simulink model "BLDC_Trapezoidal_Control"  (R2019a)
settings: Solver=VariableStepAuto  StartTime=0.0  StopTime=20  RelTol=1e-3  AbsTol=1e-3  EnableMultiTasking=on
undefined symbols (not defined in the file): sigbuilder_block
libraries: nesl_utility x14, ee_lib x12, fl_lib x8, simulink x3, powerlib_meascontrol x1
settings Model: Creator=hp  LastModifiedBy=hp
settings SolverCC: AutoScaleAbsTol=off
settings DataIOCC: LimitDataPoints=on  MaxDataPoints=10000
settings OptimizationCC: LifeSpan=inf
settings DebuggingCC: AllowSymbolicDim=off  PregeneratedLibrarySubsystemCodeDiagnostic=none  SFUnexpectedBacktrackingDiag=warning  SFNoUnconditionalDefaultTransitionDiag=warning  SFExecutionAtInitializationDiag=none  ArithmeticOperatorsInVariantConditions=warning
settings SFSimCC: SimUseLocalCustomCode=off
settings RTWCC: RTWUseLocalCustomCode=off
settings CodeAppCC: StateflowObjectComments=on
settings GRTTargetCC: TargetLangStandard=C89/C90 (ANSI)  GeneratePreprocessorConditionals=Disable all
settings ConfigComp: CovMetricSettings=dw  CovHtmlReporting=on  CovSaveCumulativeToWorkspaceVar=on  CovSaveSingleToWorkspaceVar=on  CovExternalEMLEnable=off  CovSFcnEnable=off
settings SimscapeCC: SimscapeLogType=all  SimscapeLogDataHistory=10000

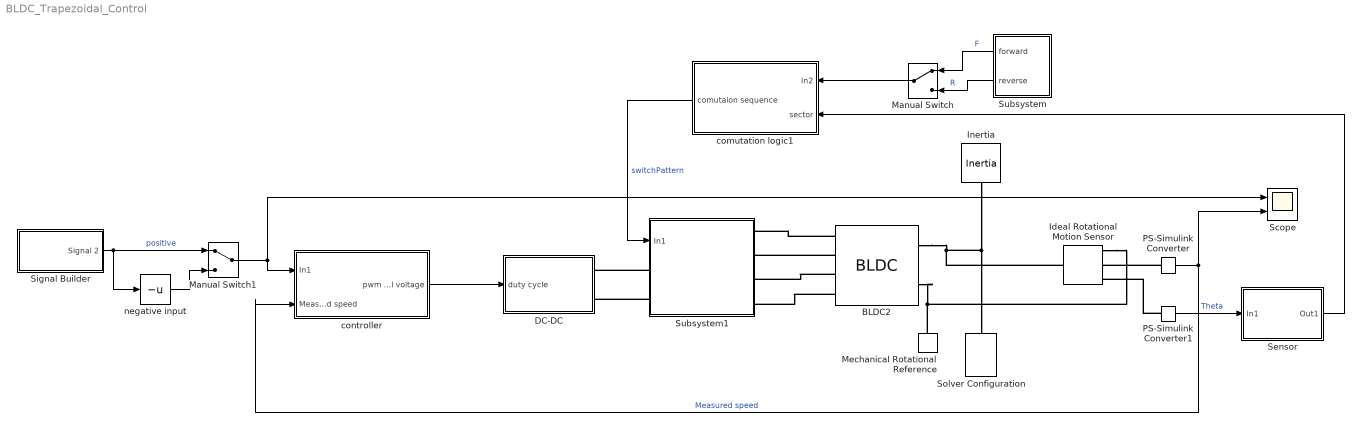
== system BLDC_Trapezoidal_Control ==
  BLDC2 : ee_lib/Electromechanical/Permanent Magnet/BLDC  rotor_param=1  pm_flux_linkage=0.5513 Wb  theta_constant=120/1 deg  emf_max=9.6 V  DphiDtheta_tab=[0, -.1528, -.1528, .1528, .1528, 0] Wb/rad  back_emf_tab=[0, -9.6, -9.6, 9.6, 9.6, 0] V  rotor_angle_tab=[0, 7.5, 22.5, 37.5, 52.5, 60] deg  w_meas=600 rpm  nPolePairs=1  stator_param=2  Ld=0.00022 H  Lq=0.00022 H  L0=0.00016 H  Ls=0.0002 H  Lm=0 H  Ms=0.00002 H  Rs=0.013 Ohm  zero_sequence=ee.enum.park.zerosequence.include  J=0.0001 kg*m^2  lam=0.2 N*m/(rad/s)  axes_param=1  i_d_specify=off  i_d_priority=None  i_d=0 A  i_d_nominal_specify=off  i_d_nominal_unit=A  i_d_nominal_value=1  i_q_specify=off  i_q_priority=None  i_q=0 A  i_q_nominal_specify=off  i_q_nominal_unit=A  i_q_nominal_value=1  torque_specify=off  torque_priority=None  torque=0 N*m  torque_nominal_specify=off  torque_nominal_unit=N*m  torque_nominal_value=1  angular_velocity_specify=off  angular_velocity_priority=High  angular_velocity=0 rpm  angular_velocity_nominal_specify=off  angular_velocity_nominal_unit=rpm  angular_velocity_nominal_value=1  angular_position_specify=off  angular_position_priority=High  angular_position=0 deg  angular_position_nominal_specify=off  angular_position_nominal_unit=deg  angular_position_nominal_value=1
      settings: SourceProductName=Simscape Electrical  SourceProductBaseCode=PS
  "DC-DC " : Subsystem
  Ideal Rotational Motion Sensor : fl_lib/Mechanical/Mechanical Sensors/Ideal Rotational Motion Sensor  offset=0 deg
  Inertia : fl_lib/Mechanical/Rotational Elements/Inertia  inertia=10 kg*m^2  w_specify=off  w_priority=High  w=0 rad/s  w_nominal_specify=off  w_nominal_unit=rad/s  w_nominal_value=1  t_specify=off  t_priority=None  t=0 N*m  t_nominal_specify=off  t_nominal_unit=N*m  t_nominal_value=1
  Manual Switch : ManualSwitch
  Manual Switch1 : ManualSwitch
  Mechanical Rotational Reference : fl_lib/Mechanical/Rotational Elements/Mechanical Rotational Reference
  PS-Simulink Converter : nesl_utility/PS-Simulink Converter  PhysicalDomain=network_engine_domain  SubClassName=ps_output  LeftPortType=input  RightPortType=output  PseudoPeriodic=off  Frequencies=[]  Unit=rpm  AffineConversion=off
  PS-Simulink Converter1 : nesl_utility/PS-Simulink Converter  PhysicalDomain=network_engine_domain  SubClassName=ps_output  LeftPortType=input  RightPortType=output  PseudoPeriodic=off  Frequencies=[]  Unit=deg  AffineConversion=off
  Scope : Scope  NumInputPorts=2
  Sensor : Subsystem
  Signal Builder : Subsystem  Tag=STV Subsys  LoadFcn=sigbuilder_block('load');  StartFcn=sigbuilder_block('start');  StopFcn=sigbuilder_block('stop');  ClipboardFcn=sigbuilder_block('clipboard');  mask(Sigbuilder block){tuvar=[0:10]}
      mask help: Simulink:masks:SigbuilderBlock_MD
      mask init:
      | if ~strcmp(get_param(bdroot(gcbh),'SimulationStatus'),'stopped') tuvar = sigbuilder_block('maskInit'); end
      settings: CopyFcn=sigbuilder_block('copy');  DeleteFcn=sigbuilder_block('delete');  ModelCloseFcn=sigbuilder_block('modelClose');  PreSaveFcn=sigbuilder_block('preSave');  PauseFcn=sigbuilder_block('pause');  ContinueFcn=sigbuilder_block('continue');  NameChangeFcn=sigbuilder_block('namechange');  OpenFcn=sigbuilder_block('open',[6 30 1012.5 447.75 ]);  CloseFcn=sigbuilder_block('close');
      mask Display: plot(0, 0, 100, 100,[2, 2, 32, 32, 2], [68, 8, 8, 68, 68],[32, 2], [38, 38], [32, 19, 2],[53, 60, 44], [32, 17, 17, 2],[16, 16, 31, 31]);txt = getActiveGroup(gcbh);text(2, 100, txt,'verticalAlignment', 'top');
  Solver Configuration : nesl_utility/Solver Configuration  PhysicalDomain=network_engine_domain  SubClassName=solver  LeftPortType=input  RightPortType=generic  Tones=[]  Harmonics=[]  SimulateNoise=off  Profile=off  UseLocalSampling=off  EnableSwitchedLinearOptims=on  FrequencyDomain=off  UseCCode=off  RelTol=0.001  AbsTol=1e-06  MinStep=1e-09  ToWorkspace=off  RevertToSquareIcSolve=off  NumHomotopyIterations=100  PhasorMode=off  PhasorModeNumHarmonics=1  DoDC=off  ResidualTolerance=1e-09  UseLocalSolver=on  LocalSolverChoice=NE_BACKWARD_EULER_ADVANCER  LocalSolverSampleTime=2e-6  DoFixedCost=on  MaxNonlinIter=3  MaxModeIter=2  LinearAlgebra=auto  EquationFormulation=NE_TIME_EF  DelaysMemoryBudget=1024  AutomaticFiltering=on  FilteringTimeConstant=0.001  PartitionStorageMethod=AS_NEEDED  PartitionMemoryBudget=1024  PartitionMethod=ROBUST
  Subsystem : Subsystem
  Subsystem1 : Subsystem
  comutation logic1 : Subsystem
  controller : Subsystem
  negative input : UnaryMinus
  wires:
  comutation logic1/1("comutaion sequence ") -> Subsystem1/1(In1)  "switchPattern"
  PS-Simulink Converter1/1 -> Sensor/1(In1)  "Theta"
  PS-Simulink Converter/1 -> Scope/2, controller/2(Measured speed)  "Measured speed"
  Sensor/1(Out1) -> comutation logic1/2(sector)
  Signal Builder/1(Signal 2) -> negative input/1, Manual Switch1/1  "positive"
  controller/1(pwm control voltage) -> "DC-DC "/1(duty cycle)
  Manual Switch/1 -> comutation logic1/1(In2)
  Subsystem/1(forward) -> Manual Switch/1  "F"
  Subsystem/2(reverse) -> Manual Switch/2  "R"
  negative input/1 -> Manual Switch1/2
  Manual Switch1/1 -> Scope/1, controller/1(In1)
  connections:
  Mechanical Rotational Reference/LConn1 -- BLDC2/RConn2 -- Ideal Rotational Motion Sensor/RConn1
  Inertia/LConn1 -- Solver Configuration/RConn1 -- Ideal Rotational Motion Sensor/LConn1 -- BLDC2/RConn1
  BLDC2/LConn1 -- Subsystem1/RConn1
  BLDC2/LConn2 -- Subsystem1/RConn2
  BLDC2/LConn3 -- Subsystem1/RConn3
  BLDC2/LConn4 -- Subsystem1/RConn4
  PS-Simulink Converter/LConn1 -- Ideal Rotational Motion Sensor/RConn2
  PS-Simulink Converter1/LConn1 -- Ideal Rotational Motion Sensor/RConn3
  Subsystem1/LConn1 -- "DC-DC "/RConn1
  Subsystem1/LConn2 -- "DC-DC "/RConn2

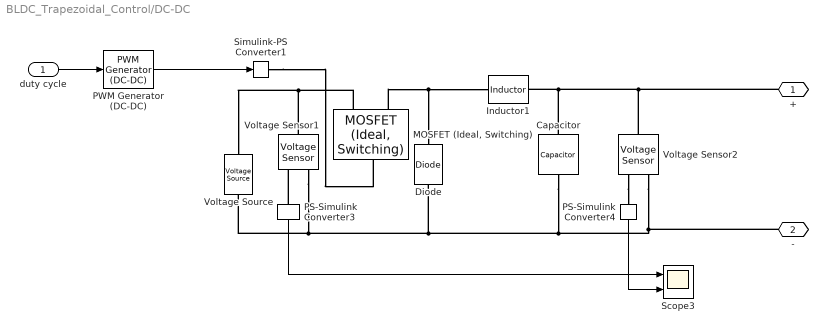
== system BLDC_Trapezoidal_Control/DC-DC  ==
  duty cycle : Inport
  Capacitor : fl_lib/Electrical/Electrical Elements/Capacitor  c=.001 F  r=.2 Ohm  g=0 1/Ohm  i_specify=off  i_priority=None  i=0 A  i_nominal_specify=off  i_nominal_unit=A  i_nominal_value=1  v_specify=off  v_priority=None  v=0 V  v_nominal_specify=off  v_nominal_unit=V  v_nominal_value=1  vc_specify=off  vc_priority=High  vc=0 V  vc_nominal_specify=off  vc_nominal_unit=V  vc_nominal_value=1
  Diode : ee_lib/Semiconductors & Converters/Diode  ModelType=ee.enum.diode.modelType.pwl  Vf=0.6 V  Ron=0.3 Ohm  Goff=1e-8 S  prmExp=ee.enum.diode.expParam.useTwo  I12=[.0137, .545] A  V12=[.6, .7] V  IS=1e-12 A  ec=1  I1=0.0137 A  V1=0.6 V  RS=0 Ohm  Tmeas=25 degC  N_series=1  N_parallel=1  Rz=0.3 Ohm  BV=inf V  C_param=ee.enum.diode.capParam.fixed  CJ=5 pF  CJ0=5 pF  VJ=1 V  Mgrad=0.5  Vvec=[.1, 10, 100] V  Cvec=[3.5, 1, .4] pF  FC=0.5  Q_param=ee.enum.diode.recoveryParam.off  iRM=-7.15 A  iF=4 A  didt=-750 A/us  trr_factor=3  trr=115 ns  Qrr=1500 s*uA  TT=50 ns  tau=100 ns  T_param=ee.enum.diode.temperatureParam.off  IS_T2=1.25e-7 A  I1_T2=0.245 A  V1_T2=0.5 V  Tmeas2=125 degC  EG_param=ee.enum.diode.egapParam.material_si  EG=1.11 eV  XTI_param=ee.enum.diode.xtiParam.pn  XTI=3  dBVdT=0 V/K  Tdevice=25 degC  i_specify=off  i_priority=None  i=0 A  i_nominal_specify=off  i_nominal_unit=A  i_nominal_value=1  v_specify=off  v_priority=None  v=0 V  v_nominal_specify=off  v_nominal_unit=V  v_nominal_value=1  i_capacitor_specify=off  i_capacitor_priority=None  i_capacitor=0 A  i_capacitor_nominal_specify=off  i_capacitor_nominal_unit=A  i_capacitor_nominal_value=1  v_capacitor_specify=off  v_capacitor_priority=None  v_capacitor=0 V  v_capacitor_nominal_specify=off  v_capacitor_nominal_unit=V  v_capacitor_nominal_value=1  power_dissipated_specify=off  power_dissipated_priority=None  power_dissipated=0 W  power_dissipated_nominal_specify=off  power_dissipated_nominal_unit=W  power_dissipated_nominal_value=1  Rth=[0, 10] K/W  thermal_mass_parameterization=ee.enum.thermalNetwork.timeconstant  thermal_mass=[0, 1] J/K  thermal_time_constant=[0, 10] s  thermal_mass_initial_temperatures=[25, 25] degC
      settings: SourceProductName=Simscape Electrical
  Inductor1 : fl_lib/Electrical/Electrical Elements/Inductor  l=.1 H  r=.1 Ohm  g=1e-9 1/Ohm  i_specify=off  i_priority=None  i=0 A  i_nominal_specify=off  i_nominal_unit=A  i_nominal_value=1  v_specify=off  v_priority=None  v=0 V  v_nominal_specify=off  v_nominal_unit=V  v_nominal_value=1  i_L_specify=off  i_L_priority=High  i_L=0 A  i_L_nominal_specify=off  i_L_nominal_unit=A  i_L_nominal_value=1
  "MOSFET (Ideal, Switching)" : ee_lib/Semiconductors & Converters/MOSFET (Ideal, Switching)  Rds=1e-4 Ohm  Goff=1e-6 1/Ohm  Vth=0.5 V  diode_param=2  diode_Vf=.1 V  diode_Ron=0.001 Ohm  diode_Goff=1e-5 1/Ohm  diode_C=50e-9 F  diode_iRM=-235 A  diode_iF=300 A  diode_idot=-50 A/us  diode_trr_param=1  diode_trr_factor=3  diode_trr=15 us  diode_Qrr=1500 s*uA  thermal_loss_option=2  Voff=300 V  Tau=1e-4 s  Tj=[298.15, 398.15] K  Iout_scalar=600 A  Eon_scalar=22.86e-3 J  Eoff_scalar=17.14e-3 J  Von_scalar=2.7 V  Iout_data=[0, 10, 50, 100, 200, 400, 600] A  Eon_data=[0, .29, 1.43, 2.86, 5.71, 13.14, 22.86; 0, .57, 2.63, 5.14, 10.29, 20.57, 30.29] * 1e-3 J  Eoff_data=[0, .21, 1.07, 2.14, 4.29, 9.86, 17.14; 0, .43, 1.97, 3.86, 7.71, 15.43, 22.71] * 1e-3 J  Von_data=[0, 1.1, 1.3, 1.45, 1.75, 2.25, 2.7; 0, 1, 1.15, 1.35, 1.7, 2.35, 3] V
      settings: SourceProductName=Simscape Electrical
  PS-Simulink Converter3 : nesl_utility/PS-Simulink Converter  PhysicalDomain=network_engine_domain  SubClassName=ps_output  LeftPortType=input  RightPortType=output  PseudoPeriodic=off  Frequencies=[]  Unit=1  AffineConversion=off
  PS-Simulink Converter4 : nesl_utility/PS-Simulink Converter  PhysicalDomain=network_engine_domain  SubClassName=ps_output  LeftPortType=input  RightPortType=output  PseudoPeriodic=off  Frequencies=[]  Unit=1  AffineConversion=off
  PWM Generator (DC-DC) : powerlib_meascontrol/Pulse & Signal Generators/PWM Generator (DC-DC)  Fsw=1000  Ts=0
      settings: SourceProductName=Simscape Electrical
  Scope3 : Scope  NumInputPorts=2
  Simulink-PS Converter1 : nesl_utility/Simulink-PS Converter  PhysicalDomain=network_engine_domain  SubClassName=ps_input  LeftPortType=input  RightPortType=output  PseudoPeriodic=off  Frequencies=[]  NoiseDistribution=none  NoiseParameters=[]  Unit=V  AffineConversion=off  FilteringAndDerivatives=provide  SimscapeFilterOrder=1  InputFilterTimeConstant=0.001  UdotUserProvided=0
  Voltage Sensor1 : fl_lib/Electrical/Electrical Sensors/Voltage Sensor
  Voltage Sensor2 : fl_lib/Electrical/Electrical Sensors/Voltage Sensor
  Voltage Source : ee_lib/Sources/Voltage Source  dc_voltage=500 V  ac_voltage=0 V  ac_shift=0 rad  ac_frequency=60 Hz  noise_mode=0  PSD=0 V^2/Hz  repeatability=1  auto_seed=387260031  user_seed=0  sample_time=1e-3 s  i_specify=off  i_priority=None  i=0 A  i_nominal_specify=off  i_nominal_unit=A  i_nominal_value=1  v_specify=off  v_priority=None  v=0 V  v_nominal_specify=off  v_nominal_unit=V  v_nominal_value=1
      settings: SourceProductName=Simscape Electrical
  + : PMIOPort  Side=Right
  - : PMIOPort  Port=2  Side=Right
  wires:
  PWM Generator (DC-DC)/1 -> Simulink-PS Converter1/1
  duty cycle/1 -> PWM Generator (DC-DC)/1
  PS-Simulink Converter4/1 -> Scope3/2
  PS-Simulink Converter3/1 -> Scope3/1
  connections:
  "MOSFET (Ideal, Switching)"/RConn1 -- Voltage Source/LConn1 -- Voltage Sensor1/LConn1
  Voltage Source/RConn1 -- Voltage Sensor2/RConn2 -- -/RConn1 -- Capacitor/RConn1 -- Diode/LConn1 -- Voltage Sensor1/RConn2
  Simulink-PS Converter1/RConn1 -- "MOSFET (Ideal, Switching)"/LConn1
  "MOSFET (Ideal, Switching)"/RConn2 -- Inductor1/LConn1 -- Diode/RConn1
  Capacitor/LConn1 -- +/RConn1 -- Voltage Sensor2/LConn1 -- Inductor1/RConn1
  Voltage Sensor2/RConn1 -- PS-Simulink Converter4/LConn1
  PS-Simulink Converter3/LConn1 -- Voltage Sensor1/RConn1

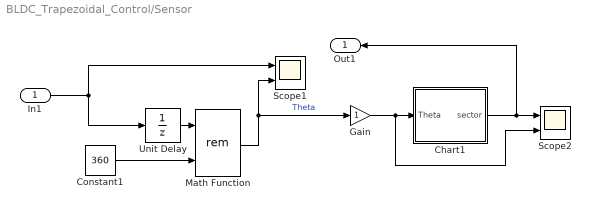
== system BLDC_Trapezoidal_Control/Sensor ==
  In1 : Inport
  Chart1 : Stateflow chart  BlockKeywords=__PRM__SERIALIZED__DATA__:Stateflow Chart,Stateflow Diagram  TreatAsAtomicUnit=on
  Constant1 : Constant  Value=360
  Gain : Gain
  Math Function : Math  Operator=rem  SaturateOnIntegerOverflow=on
  Scope1 : Scope  NumInputPorts=2
  Scope2 : Scope  NumInputPorts=2
  Unit Delay : UnitDelay  SampleTime=-1  HasFrameUpgradeWarning=on
  Out1 : Outport
  wires:
  Chart1/1(sector) -> Out1/1, Scope2/1
  Constant1/1 -> Math Function/2
  Unit Delay/1 -> Math Function/1
  In1/1 -> Scope1/1, Unit Delay/1
  Math Function/1 -> Gain/1, Scope1/2  "Theta"
  Gain/1 -> Chart1/1(Theta), Scope2/2

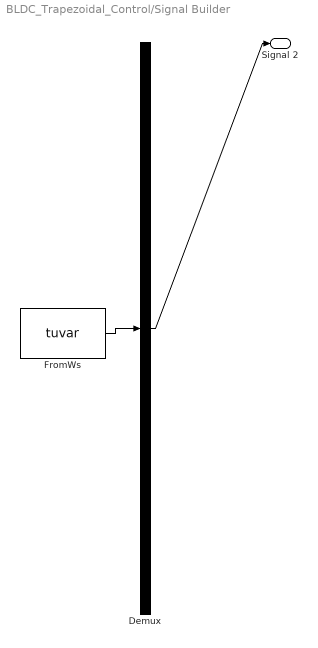
== system BLDC_Trapezoidal_Control/Signal Builder ==
  Demux : Demux  Tag=STV Demux  Outputs=1
  FromWs : FromWorkspace  Tag=STV FromWs  VariableName=tuvar  SampleTime=0
      SigBuilderData=|
      | common.afterFinalStr = 'Extrapolate'
      | common.sampleTime = 0
      | dataSet.timeRange = [0 15]
      | dataSet.name = 'Group 1'
      | sbobj.Groups.Name = 'Group 1'
      | sbobj.Groups.Signals.Name = 'Signal 2'
      | sbobj.Groups.Signals.XData = [0 1.66666666667 3.33333333333 5 6.66666666667 8.33333333333 10 11.6666666667 13.3333333333 15]
      | sbobj.Groups.Signals.YData = [0 270 510 520 780 1000 1000 1380 1500 1510]
      | sbobj.Groups.TimeRange = [0 15]
  Signal 2 : Outport  Tag=STV Outport
  wires:
  FromWs/1 -> Demux/1
  Demux/1 -> Signal 2/1

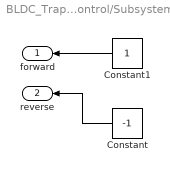
== system BLDC_Trapezoidal_Control/Subsystem ==
  Constant : Constant  Value=-1
  Constant1 : Constant
  forward : Outport
  reverse : Outport  Port=2
  wires:
  Constant/1 -> reverse/1
  Constant1/1 -> forward/1

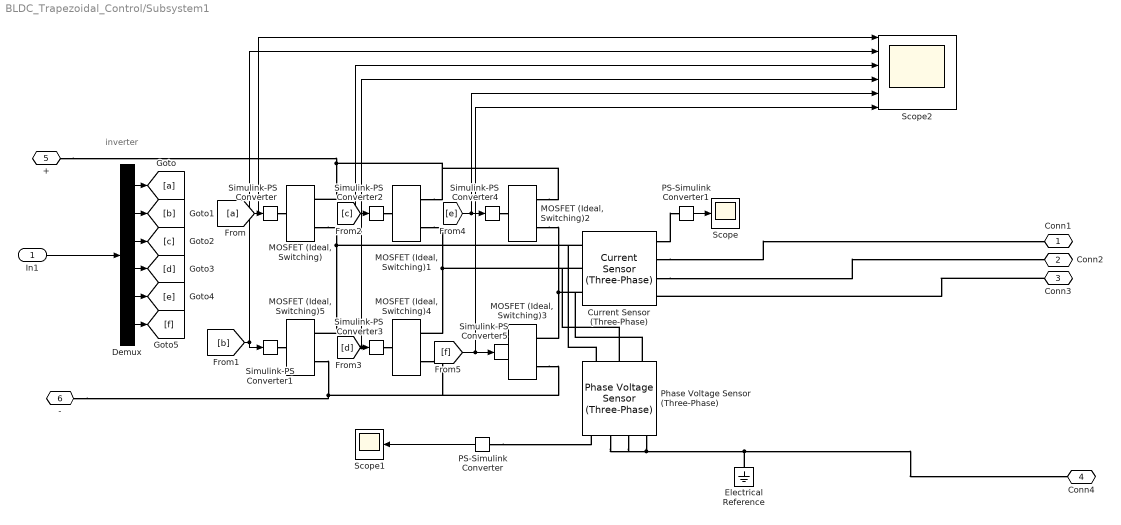
== system BLDC_Trapezoidal_Control/Subsystem1 ==
  note: inverter
  In1 : Inport
  Current Sensor (Three-Phase) : ee_lib/Sensors & Transducers/Current Sensor (Three-Phase)
      settings: SourceProductName=Simscape Electrical
  Demux : Demux  Outputs=6
  Electrical Reference : fl_lib/Electrical/Electrical Elements/Electrical Reference
  MOSFET (Ideal, Switching){,1..5} (6 alike) : ee_lib/Semiconductors & Converters/MOSFET (Ideal, Switching)  Rds=0.01 Ohm  Goff=1e-6 1/Ohm  Vth=.5 V  diode_param=2  diode_Vf=.1 V  diode_Ron=0.001 Ohm  diode_Goff=1e-5 1/Ohm  diode_C=50e-9 F  diode_iRM=-235 A  diode_iF=300 A  diode_idot=-50 A/us  diode_trr_param=1  diode_trr_factor=3  diode_trr=15 us  diode_Qrr=1500 s*uA  thermal_loss_option=2  Voff=300 V  Tau=1e-4 s  Tj=[298.15, 398.15] K  Iout_scalar=600 A  Eon_scalar=22.86e-3 J  Eoff_scalar=17.14e-3 J  Von_scalar=2.7 V  Iout_data=[0, 10, 50, 100, 200, 400, 600] A  Eon_data=[0, .29, 1.43, 2.86, 5.71, 13.14, 22.86; 0, .57, 2.63, 5.14, 10.29, 20.57, 30.29] * 1e-3 J  Eoff_data=[0, .21, 1.07, 2.14, 4.29, 9.86, 17.14; 0, .43, 1.97, 3.86, 7.71, 15.43, 22.71] * 1e-3 J  Von_data=[0, 1.1, 1.3, 1.45, 1.75, 2.25, 2.7; 0, 1, 1.15, 1.35, 1.7, 2.35, 3] V
      settings: SourceProductName=Simscape Electrical
  PS-Simulink Converter : nesl_utility/PS-Simulink Converter  PhysicalDomain=network_engine_domain  SubClassName=ps_output  LeftPortType=input  RightPortType=output  PseudoPeriodic=off  Frequencies=[]  Unit=1  AffineConversion=off
  PS-Simulink Converter1 : nesl_utility/PS-Simulink Converter  PhysicalDomain=network_engine_domain  SubClassName=ps_output  LeftPortType=input  RightPortType=output  PseudoPeriodic=off  Frequencies=[]  Unit=1  AffineConversion=off
  Phase Voltage Sensor (Three-Phase) : ee_lib/Sensors & Transducers/Phase Voltage Sensor (Three-Phase)
      settings: SourceProductName=Simscape Electrical  SourceProductBaseCode=PS
  Scope : Scope
  Scope1 : Scope
  Scope2 : Scope  NumInputPorts=6
  Simulink-PS Converter{,1..5} (6 alike) : nesl_utility/Simulink-PS Converter  PhysicalDomain=network_engine_domain  SubClassName=ps_input  LeftPortType=input  RightPortType=output  PseudoPeriodic=off  Frequencies=[]  NoiseDistribution=none  NoiseParameters=[]  Unit=1  AffineConversion=off  FilteringAndDerivatives=provide  SimscapeFilterOrder=1  InputFilterTimeConstant=0.001  UdotUserProvided=0
  Conn1 : PMIOPort  Side=Right
  Conn2 : PMIOPort  Port=2  Side=Right
  Conn3 : PMIOPort  Port=3  Side=Right
  Conn4 : PMIOPort  Port=4  Side=Right
  + : PMIOPort  Port=5  Side=Left
  - : PMIOPort  Port=6  Side=Left
  wires:
  [c] -> Scope2/3, Simulink-PS Converter2/1
  PS-Simulink Converter1/1 -> Scope/1
  [d] -> Simulink-PS Converter3/1, Scope2/4
  Demux/5 -> [e]
  Demux/3 -> [c]
  Demux/2 -> [b]
  Demux/4 -> [d]
  [f] -> Scope2/6, Simulink-PS Converter5/1
  [e] -> Scope2/5, Simulink-PS Converter4/1
  Demux/1 -> [a]
  Demux/6 -> [f]
  PS-Simulink Converter/1 -> Scope1/1
  [b] -> Scope2/2, Simulink-PS Converter1/1
  In1/1 -> Demux/1
  [a] -> Scope2/1, Simulink-PS Converter/1
  connections:
  "MOSFET (Ideal, Switching)2"/RConn1 -- "MOSFET (Ideal, Switching)1"/RConn1 -- +/RConn1 -- "MOSFET (Ideal, Switching)"/RConn1
  Simulink-PS Converter4/RConn1 -- "MOSFET (Ideal, Switching)2"/LConn1
  Electrical Reference/LConn1 -- Conn4/RConn1 -- Phase Voltage Sensor (Three-Phase)/RConn2 -- Phase Voltage Sensor (Three-Phase)/RConn3 -- Phase Voltage Sensor (Three-Phase)/RConn4
  "MOSFET (Ideal, Switching)1"/RConn2 -- Phase Voltage Sensor (Three-Phase)/LConn2 -- Current Sensor (Three-Phase)/LConn2 -- "MOSFET (Ideal, Switching)4"/RConn1
  "MOSFET (Ideal, Switching)"/RConn2 -- Phase Voltage Sensor (Three-Phase)/LConn1 -- Current Sensor (Three-Phase)/LConn1 -- "MOSFET (Ideal, Switching)5"/RConn1
  Simulink-PS Converter5/RConn1 -- "MOSFET (Ideal, Switching)3"/LConn1
  Simulink-PS Converter1/RConn1 -- "MOSFET (Ideal, Switching)5"/LConn1
  Current Sensor (Three-Phase)/RConn1 -- PS-Simulink Converter1/LConn1
  "MOSFET (Ideal, Switching)5"/RConn2 -- -/RConn1 -- "MOSFET (Ideal, Switching)3"/RConn2 -- "MOSFET (Ideal, Switching)4"/RConn2
  Current Sensor (Three-Phase)/RConn2 -- Conn1/RConn1
  Simulink-PS Converter2/RConn1 -- "MOSFET (Ideal, Switching)1"/LConn1
  Simulink-PS Converter3/RConn1 -- "MOSFET (Ideal, Switching)4"/LConn1
  "MOSFET (Ideal, Switching)2"/RConn2 -- Phase Voltage Sensor (Three-Phase)/LConn3 -- Current Sensor (Three-Phase)/LConn3 -- "MOSFET (Ideal, Switching)3"/RConn1
  PS-Simulink Converter/LConn1 -- Phase Voltage Sensor (Three-Phase)/RConn1
  Simulink-PS Converter/RConn1 -- "MOSFET (Ideal, Switching)"/LConn1
  Current Sensor (Three-Phase)/RConn3 -- Conn2/RConn1
  Conn3/RConn1 -- Current Sensor (Three-Phase)/RConn4

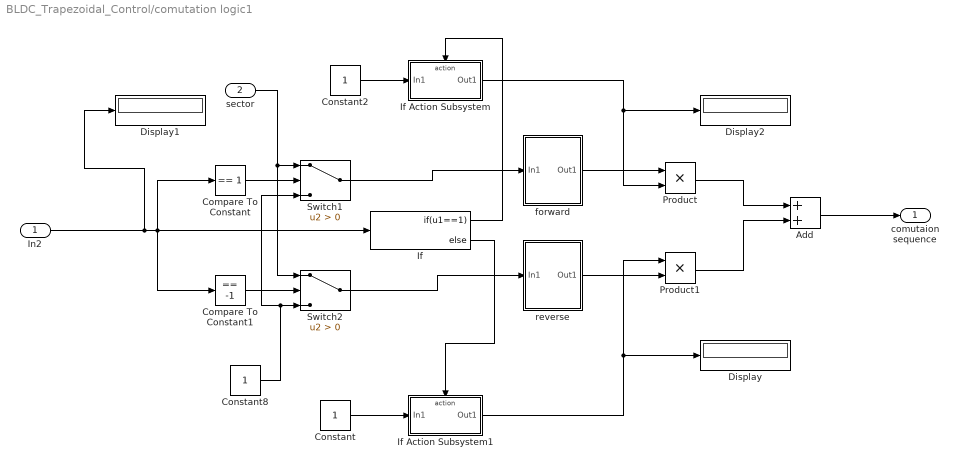
== system BLDC_Trapezoidal_Control/comutation logic1 ==
  In2 : Inport
  sector : Inport  Port=2
  Add : Sum
  Compare To Constant : simulink/Logic and Bit Operations/Compare To Constant  relop===  const=1  OutDataTypeStr=boolean
  Compare To Constant1 : simulink/Logic and Bit Operations/Compare To Constant  relop===  const=-1  OutDataTypeStr=boolean
  Constant : Constant
  Constant2 : Constant
  Constant8 : Constant
  Display : Display
  Display1 : Display
  Display2 : Display
  If : If  IfExpression=u1==1
  If Action Subsystem : Subsystem  TreatAsAtomicUnit=on
  If Action Subsystem1 : Subsystem  TreatAsAtomicUnit=on
  Product : Product
  Product1 : Product
  Switch1 : Switch  Criteria=u2 > Threshold
  Switch2 : Switch  Criteria=u2 > Threshold
  forward : Subsystem
  reverse : Subsystem
  "comutaion sequence " : Outport
  wires:
  In2/1 -> Display1/1, Compare To Constant/1, If/1, Compare To Constant1/1
  Compare To Constant/1 -> Switch1/2
  Compare To Constant1/1 -> Switch2/2
  sector/1 -> Switch2/1, Switch1/1
  Constant8/1 -> Switch1/3, Switch2/3
  Switch1/1 -> forward/1(In1)
  Switch2/1 -> reverse/1(In1)
  Add/1 -> "comutaion sequence "/1
  If/2 -> If Action Subsystem1/Action
  If/1 -> If Action Subsystem/Action
  forward/1(Out1) -> Product/1
  reverse/1(Out1) -> Product1/2
  Product1/1 -> Add/2
  Product/1 -> Add/1
  If Action Subsystem/1(Out1) -> Display2/1, Product/2
  If Action Subsystem1/1(Out1) -> Product1/1, Display/1
  Constant/1 -> If Action Subsystem1/1(In1)
  Constant2/1 -> If Action Subsystem/1(In1)

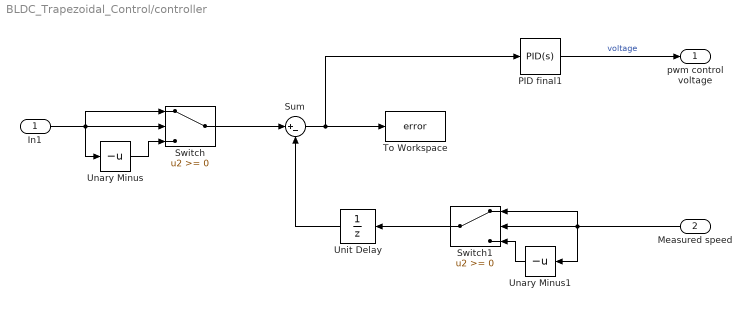
== system BLDC_Trapezoidal_Control/controller ==
  In1 : Inport
  Measured speed : Inport  Port=2
  PID final1 : simulink/Continuous/PID Controller  Controller=PID  Form=Parallel  TimeDomain=Continuous-time  SampleTime=-1  IntegratorMethod=Forward Euler  FilterMethod=Forward Euler  ControllerParametersSource=internal  P=.1  I=.03  D=.01  UseFilter=on  N=100  TunerSelectOption=Transfer Function Based (PID Tuner App)  InitialConditionSource=internal  InitialConditionForIntegrator=0  InitialConditionForFilter=0  DifferentiatorICPrevScaledInput=0  ExternalReset=none  TrackingMode=off  Kt=1  LimitOutput=on  UpperSaturationLimit=1  LowerSaturationLimit=0  LinearizeAsGain=on  AntiWindupMode=clamping  Kb=1  POutMin=[]  POutMax=[]  IOutMin=[]  IOutMax=[]  DOutMin=[]  DOutMax=[]  NOutMin=[]  NOutMax=[]  SumOutMin=[]  SumOutMax=[]  SaturationOutMin=[]  SaturationOutMax=[]  PParamMin=[]  PParamMax=[]  IParamMin=[]  IParamMax=[]  DParamMin=[]  DParamMax=[]  NParamMin=[]  NParamMax=[]  KbParamMin=[]  KbParamMax=[]  KtParamMin=[]  KtParamMax=[]  KbOutMin=[]  KbOutMax=[]  KtOutMin=[]  KtOutMax=[]  IntegratorOutMin=[]  IntegratorOutMax=[]  FilterOutMin=[]  FilterOutMax=[]  SumI1OutMin=[]  SumI1OutMax=[]  SumI2OutMin=[]  SumI2OutMax=[]  SumI3OutMin=[]  SumI3OutMax=[]  SumI4OutMin=[]  SumI4OutMax=[]  SumDOutMin=[]  SumDOutMax=[]  DifferentiatorOutMin=[]  DifferentiatorOutMax=[]  FilterDiffOutCoefMin=[]  FilterDiffOutCoefMax=[]  ReciprocalOutMin=[]  ReciprocalOutMax=[]  SumDenOutMin=[]  SumDenOutMax=[]  SumNumOutMin=[]  SumNumOutMax=[]  DivideOutMin=[]  DivideOutMax=[]  IntegratorContinuousStateAttributes=''  IntegratorStateMustResolveToSignalObject=off  IntegratorRTWStateStorageClass=Auto  FilterContinuousStateAttributes=''  FilterStateMustResolveToSignalObject=off  FilterRTWStateStorageClass=Auto  ParallelPVariant=InternalParameters  IdealPVariant=Disabled  IVariant=InternalParameters  DVariant=InternalParameters  IntegratorVariant=Continuous  SatVariant=Enabled  AWVariant=ContClampingParallel  PCopyVariant=Disabled  TRVariant=Disabled  FdbkBlocksVariant=Forward  IdealPFdbkVariant=Disabled  SatFdbkVariant=Disabled  DerivativeFilterVariant=ContFilter  NVariant=InternalParameters  NCopyVariant=Disabled  FilterICVariant=InternalICsFilter  IntegratorICVariant=InternalICs  ExternalResetVariant=Disabled  TRSumVariant=Passthrough  SumFdbkVariant=Disabled  SumVariant=Sum_PID
  Sum : Sum  Inputs=|+-
  Switch : Switch
  Switch1 : Switch
  To Workspace : ToWorkspace  VariableName=error  SampleTime=-1
  Unary Minus : UnaryMinus
  Unary Minus1 : UnaryMinus
  Unit Delay : UnitDelay  SampleTime=-1  HasFrameUpgradeWarning=on
  pwm control voltage : Outport
  wires:
  Unit Delay/1 -> Sum/2
  PID final1/1 -> pwm control voltage/1  "voltage"
  Sum/1 -> PID final1/1, To Workspace/1
  Measured speed/1 -> Switch1/1, Switch1/2, Unary Minus1/1
  Switch1/1 -> Unit Delay/1
  In1/1 -> Switch/1, Switch/2, Unary Minus/1
  Unary Minus/1 -> Switch/3
  Switch/1 -> Sum/1
  Unary Minus1/1 -> Switch1/3

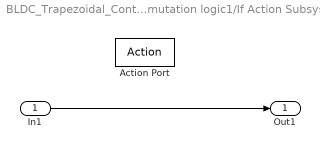
== system BLDC_Trapezoidal_Control/comutation logic1/If Action Subsystem ==
  In1 : Inport
  Action Port : ActionPort  InitializeStates=reset  ActionPortLabel=if(u1==1)
  Out1 : Outport
  wires:
  In1/1 -> Out1/1

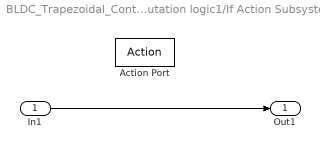
== system BLDC_Trapezoidal_Control/comutation logic1/If Action Subsystem1 ==
  In1 : Inport
  Action Port : ActionPort  ActionPortLabel=else
  Out1 : Outport
  wires:
  In1/1 -> Out1/1

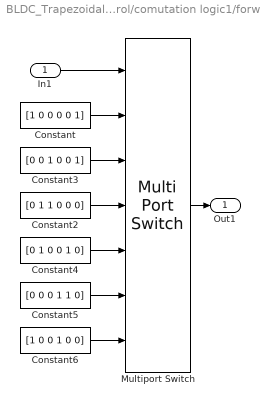
== system BLDC_Trapezoidal_Control/comutation logic1/forward ==
  In1 : Inport
  Constant : Constant  Value=[1 0 0 0 0 1]
  Constant2 : Constant  Value=[0 1 1 0 0 0]
  Constant3 : Constant  Value=[0 0 1 0 0 1]
  Constant4 : Constant  Value=[0 1 0 0 1 0]
  Constant5 : Constant  Value=[0 0 0 1 1 0]
  Constant6 : Constant  Value=[1 0 0 1 0 0]
  Multiport Switch : MultiPortSwitch  Inputs=6
  Out1 : Outport
  wires:
  Constant5/1 -> Multiport Switch/6
  Constant2/1 -> Multiport Switch/4
  Constant/1 -> Multiport Switch/2
  Constant4/1 -> Multiport Switch/5
  Constant3/1 -> Multiport Switch/3
  In1/1 -> Multiport Switch/1
  Constant6/1 -> Multiport Switch/7
  Multiport Switch/1 -> Out1/1

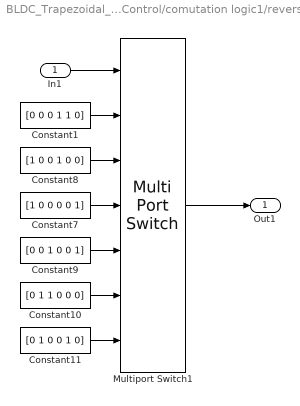
== system BLDC_Trapezoidal_Control/comutation logic1/reverse ==
  In1 : Inport
  Constant1 : Constant  Value=[0 0 0 1 1 0]
  Constant10 : Constant  Value=[0 1 1 0 0 0]
  Constant11 : Constant  Value=[0 1 0 0 1 0]
  Constant7 : Constant  Value=[1 0 0 0 0 1]
  Constant8 : Constant  Value=[1 0 0 1 0 0]
  Constant9 : Constant  Value=[0 0 1 0 0 1]
  Multiport Switch1 : MultiPortSwitch  Inputs=6
  Out1 : Outport
  wires:
  Constant11/1 -> Multiport Switch1/7
  Constant10/1 -> Multiport Switch1/6
  Constant9/1 -> Multiport Switch1/5
  Constant7/1 -> Multiport Switch1/4
  Constant1/1 -> Multiport Switch1/2
  Constant8/1 -> Multiport Switch1/3
  Multiport Switch1/1 -> Out1/1
  In1/1 -> Multiport Switch1/1

== stateflow chart BLDC_Trapezoidal_Control/Sensor/Chart1 ==
  state sector6
    sector=6;
  state sector5
    sector=5;
  state sector1
    sector=1;
  state sector4
    sector=4;
  note: Commutation
      | Logic
  state sector2
    sector=2;
  state sector3
    sector=3;
  sector6 -> sector1 [order 1] : [0<=Theta&&Theta<60]
  sector4 -> sector5 [order 1] : [240<=Theta&&Theta<300]
  sector5 -> sector6 [order 1] : [300<=Theta&&Theta<360]
  sector5 -> sector4 [order 2] : [-180<Theta&&Theta<=-120]
  sector1 -> sector6 [order 2] : [-60<Theta&&Theta<=0]
  sector6 -> sector5 [order 2] : [-120<Theta&&Theta<=-60]
  (default) -> sector1
  sector1 -> sector2 [order 1] : [60<=Theta&&Theta<120]
  sector2 -> sector1 [order 2] : [-360<Theta&&Theta<=-300]
  sector3 -> sector4 [order 1] : [180<=Theta&&Theta<240]
  sector4 -> sector3 [order 2] : [-240<Theta&&Theta<=-180]
  sector3 -> sector2 [order 2] : [-300<Theta&&Theta<=-240]
  sector2 -> sector3 [order 1] : [120<=Theta&&Theta<180]
  data: sector output; Theta input
